simulink model "ModeSwitching"  (R2024a)
settings: Solver=FixedStepAuto  StartTime=0.0  StopTime=20  FixedStep=0.0005  RelTol=1e-3
values from neighbouring files (symbols this model uses):
  efficiency_map = efficiency_map / 100    [ModeSwitching_para.m]
  radius = 0.527    [ModeSwitching_para.m]
  s_thr = 0.2    [ModeSwitching_para.m]
  speed_rpm = [500,1000,1500,2000,2500,3000,3500,4000,4500,5000,5500,6000,6500,7000,7500,8000,8500,9000,9500,10000,10500,11000,11500,12000]    [ModeSwitching_para.m]
  torque_nm = [-600	-590	-580	-570	-560	-550	-540	-530	-520	-510	-500	-490	-480	-470	-460	-450	-440	-430	-420	-410	-400	-390	-380	-370	-360	-350	-340	-330	-320	-310	-300	-290	-280	-270	-260	-250	-240	-230	-220	-210	-200	-190	-180	-170	-160	-150	-140	-130	-120	-110	-100	-90	-80	-70	-60	-50	-40	-30	-20	-10	10	20	30	40	50	60	70	80	90	100	110	120	130	140	150	160	170	180	190	200	210	220	230	240	250	260	270	280	290	3 ...(+123 chars)    [ModeSwitching_para.m]
  v_min_s = 0.7    [ModeSwitching_para.m]
libraries: Solver_SF x1
(part 1 of 2)
settings Model: Creator=pan18  LastModifiedBy=pan18

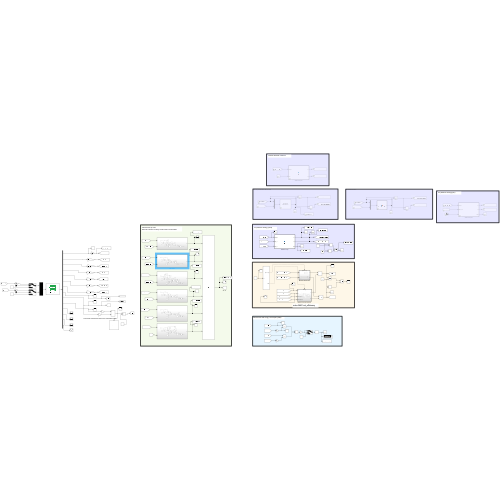
[thumbnail: Simulink's stored preview of the top-level diagram]
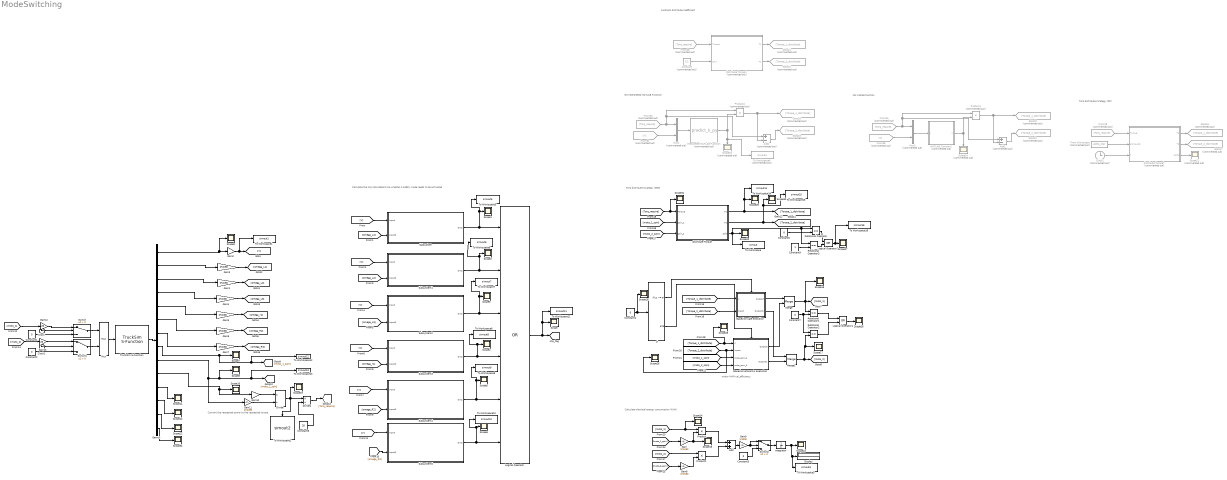
== system ModeSwitching ==
  note: NN matlab function
  note: NN Interpreted MATLAB Function
  note: Convert the requested power to the requested torque.
  note: Torq distribute strategy (GGS)
  note: Calculate the slip ratio
      | Determine whether a safety mode needs to be activated
  note: Calculate the total energy consumption (kWh)
  note: motor MAP-cal_efficiency
  note: constant distribute coefficient
  note: Torq distribute strategy (DP)
  Add : Sum
  Add1 : Sum  Commented=on  Inputs=+-
  Add2 : Sum  Commented=on  Inputs=+-
  Based on economic execution : Subsystem  TreatAsAtomicUnit=on
  Based on safe execution : Subsystem  TreatAsAtomicUnit=on
  Clock : Clock
  Clock1 : Clock
  Clock2 : Clock  Commented=on
  Constant : Constant  Commented=on  Value=0.2
  Constant{1..5,7} (6 alike) : Constant  Value=0
  Constant6 : Constant  Value=20
  Constant9 : Constant
  Demux : Demux  Outputs=14
  Display : Display
  Divide : Product  Inputs=*/
  Divide1 : Product  Inputs=*/
  From Workspace : FromWorkspace  Commented=on  VariableName=alpha_star
  From{28..30,34} (4 alike) : From  Commented=on  GotoTag=Torq_require
  From31 : From  Commented=on  GotoTag=V
  From35 : From  Commented=on  GotoTag=V
  Gain{,1,3..8,11} (9 alike) : Gain  Gain=2*pi/60
  Gain10 : Gain  Gain=1000
  Gain12 : Gain  Gain=20
  Gain13 : Gain  Gain=20
  Gain2 : Gain  Gain=1/3.6
  Gain9 : Gain  Gain=1/1000
  Goto{14,16,18,20} (4 alike) : Goto  Commented=on  GotoTag=Torque_1_distribute
  Goto{15,17,19,21} (4 alike) : Goto  Commented=on  GotoTag=Torque_2_distribute
  If : If  IfExpression=u1 ~= 0
  Integrator : Integrator
  Interpreted MATLAB Function : MATLABFcn  Commented=on  MATLABFcn=predict_k_py
  Logical Operator : Logic  Operator=OR  Inputs=6  AllPortsSameDT=off  OutDataTypeStr=boolean
  Logical Operator1 : Logic  Operator=OR  AllPortsSameDT=off  OutDataTypeStr=boolean
  Logical Operator2 : Logic  Operator=OR  AllPortsSameDT=off  OutDataTypeStr=boolean
  MATLAB Function1 : MATLAB Function  Commented=on  TreatAsAtomicUnit=on
  Merge : Merge
  Merge1 : Merge
  Mux : Mux  Inputs=2
  Mux1 : Mux  Commented=on  Inputs=2
  Mux3 : Mux  Commented=on  Inputs=2
  Product : Product
  Product1 : Product
  Product2 : Product  Commented=on
  Product4 : Product  Commented=on
  Relational Operator{,1..3} (4 alike) : RelationalOperator  Operator===  OutDataTypeStr=boolean  RndMeth=Simplest  InputSameDT=off
  Scope{,1..20,22,25..32} (30 alike) : Scope
  Scope21 : Scope  Commented=on
  Scope23 : Scope  Commented=on
  Scope24 : Scope  Commented=on
  Subsystem : Subsystem
  Subsystem1 : Subsystem
  Subsystem2 : Subsystem
  Subsystem3 : Subsystem
  Subsystem4 : Subsystem
  Subsystem6 : Subsystem
  Switch : Switch  Criteria=u2 > Threshold  SaturateOnIntegerOverflow=off  InputSameDT=off
  Switch1 : Switch  Criteria=u2 > Threshold  SaturateOnIntegerOverflow=off  InputSameDT=off
  Switch2 : Switch  Criteria=u2 > Threshold  SaturateOnIntegerOverflow=off  InputSameDT=off
  To Workspace : ToWorkspace  VariableName=simout  SaveFormat=Timeseries  SampleTime=-1
  To Workspace1 : ToWorkspace  VariableName=simout1  SaveFormat=Timeseries  SampleTime=-1
  To Workspace10 : ToWorkspace  VariableName=simout10  SaveFormat=Timeseries  SampleTime=-1
  To Workspace11 : ToWorkspace  VariableName=simout11  SaveFormat=Timeseries  SampleTime=-1
  To Workspace12 : ToWorkspace  VariableName=simout12  SaveFormat=Timeseries  SampleTime=-1
  To Workspace13 : ToWorkspace  VariableName=simout13  SaveFormat=Timeseries  SampleTime=-1
  To Workspace14 : ToWorkspace  VariableName=simout14  SaveFormat=Timeseries  SampleTime=-1
  To Workspace15 : ToWorkspace  VariableName=simout15  SaveFormat=Timeseries  SampleTime=-1
  To Workspace16 : ToWorkspace  VariableName=simout16  SaveFormat=Timeseries  SampleTime=-1
  To Workspace2 : ToWorkspace  VariableName=simout2  SaveFormat=Timeseries  SampleTime=-1
  To Workspace3 : ToWorkspace  VariableName=simout3  SaveFormat=Timeseries  SampleTime=-1
  To Workspace4 : ToWorkspace  Commented=on  VariableName=simout4  SaveFormat=Timeseries  SampleTime=-1
  To Workspace5 : ToWorkspace  VariableName=simout5  SaveFormat=Timeseries  SampleTime=-1
  To Workspace6 : ToWorkspace  VariableName=simout6  SaveFormat=Timeseries  SampleTime=-1
  To Workspace7 : ToWorkspace  VariableName=simout7  SaveFormat=Timeseries  SampleTime=-1
  To Workspace8 : ToWorkspace  VariableName=simout8  SaveFormat=Timeseries  SampleTime=-1
  To Workspace9 : ToWorkspace  VariableName=simout9  SaveFormat=Timeseries  SampleTime=-1
  TruckSim S-Function : Solver_SF/TruckSim S-Function  Priority=1  SIMFILE=simfile.sim  Run_RTs=off  vs_state_ind=Run  StopMode_ind=Vehicle Model
      settings: SourceProductName=TruckSim S-Function
  distribute Torque : MATLAB Function  TreatAsAtomicUnit=on
  distribute Torque1 : MATLAB Function  Commented=on  TreatAsAtomicUnit=on
  distribute Torque2 : MATLAB Function  Commented=on  TreatAsAtomicUnit=on
  wires:
  TruckSim S-Function/1 -> Demux/1
  Demux/1 -> Scope9/1, Gain2/1
  Demux/3 -> Gain1/1
  Gain2/1 -> To Workspace1/1, [V]
  Gain1/1 -> [omega_L2]
  Gain3/1 -> [omega_L1]
  Demux/2 -> Gain3/1
  Demux/4 -> Gain4/1
  Gain4/1 -> [omega_L3]
  Demux/5 -> Gain5/1
  Demux/6 -> Gain6/1
  Demux/7 -> Gain7/1
  Gain5/1 -> [omega_r1]
  Gain6/1 -> [omega_R2]
  Gain7/1 -> [omega_R3]
  [V] -> Subsystem/1(Inport)
  [omega_L1] -> Subsystem/2(Inport2)
  [omega_L2] -> Subsystem1/2(Inport2)
  [V] -> Subsystem1/1(Inport)
  [V] -> Subsystem2/1(Inport)
  [omega_L3] -> Subsystem2/2(Inport2)
  [V] -> Subsystem3/1(Inport)
  [V] -> Subsystem4/1(Inport)
  [omega_r1] -> Subsystem3/2(Inport2)
  [omega_R2] -> Subsystem4/2(Inport2)
  [V] -> Subsystem6/1(Inport)
  [omega_R3] -> Subsystem6/2(Inport2)
  Subsystem/1(Out1) -> To Workspace5/1, Scope1/1, Logical Operator/1
  Subsystem1/1(Out1) -> To Workspace6/1, Scope2/1, Logical Operator/2
  Subsystem3/1(Out1) -> To Workspace8/1, Scope4/1, Logical Operator/4
  Subsystem4/1(Out1) -> To Workspace9/1, Scope5/1, Logical Operator/5
  Logical Operator/1 -> To Workspace11/1, Scope/1, [Slip_tag]
  Subsystem2/1(Out1) -> To Workspace7/1, Scope3/1, Logical Operator/3
  Subsystem6/1(Out1) -> To Workspace10/1, Scope6/1, Logical Operator/6
  Constant1/1 -> Switch/3
  Constant2/1 -> Switch1/3
  Clock/1 -> Switch/2
  Clock1/1 -> Switch1/2
  [moto_1] -> Gain12/1
  [moto_2] -> Gain13/1
  If/1 -> Based on safe execution/Action
  If/2 -> Based on economic execution/Action
  Based on safe execution/1(Outport) -> Merge/1
  Based on economic execution/1(Outport) -> Merge/2
  Based on safe execution/2(Outport1) -> Merge1/1
  Based on economic execution/2(Outport1) -> Merge1/2
  Merge/1 -> Scope16/1, Relational Operator1/1, [moto_1]
  Merge1/1 -> Relational Operator2/2, Scope17/1, [moto_2]
  Demux/9 -> To Workspace13/1, [moto_2_spin], Scope8/1, Gain11/1
  [moto_1_spin] -> distribute Torque/2(spin_1)
  distribute Torque/1(T1) -> To Workspace14/1, Scope29/1, [Torque_1_distribute]
  distribute Torque/2(T2) -> Scope30/1, To Workspace15/1, [Torque_2_distribute]
  Demux/10 -> Gain10/1, Scope10/1
  Demux/11 -> Scope11/1
  Demux/12 -> Scope12/1
  [Torq_require] -> Scope31/1, distribute Torque/1(Torque)
  [Torque_1_distribute] -> Scope25/1, Based on economic execution/1(u)
  [Torque_2_distribute] -> Scope26/1, Based on economic execution/2(Inport)
  [moto_1_spin] -> Based on economic execution/3(moto_spin_1)
  [moto_2_spin] -> Based on economic execution/4(moto_spin_2)
  [Torque_2_distribute] -> Based on safe execution/2(Inport)
  [Torque_1_distribute] -> Based on safe execution/1(u)
  Switch1/1 -> Mux/2
  Switch/1 -> Mux/1
  [moto_1_spin] -> Gain/1
  [moto_2_spin] -> Gain8/1
  [moto_1] -> Scope14/1, Product/1
  Gain/1 -> Scope15/1, Product/2
  [moto_2] -> Product1/1
  Gain8/1 -> Product1/2
  Product/1 -> Add/1
  Product1/1 -> Add/2
  Add/1 -> Gain9/1
  Integrator/1 -> To Workspace3/1, Display/1, Scope13/1
  [moto_2_spin] -> distribute Torque/3(spin_2)
  Gain10/1 -> Divide/1
  Divide/1 -> Divide1/1, To Workspace2/1, Scope19/1
  Gain11/1 -> Divide/2
  Constant/1 -> distribute Torque1/2(split)
  distribute Torque1/1(T1) -> Goto14/1
  From28/1 -> distribute Torque1/1(Torque)
  distribute Torque1/2(T2) -> Goto15/1
  Constant4/1 -> Scope18/1, If/1
  distribute Torque/3(split) -> Relational Operator3/1, Relational Operator/1, Scope20/1, To Workspace/1
  Mux/1 -> TruckSim S-Function/1
  distribute Torque2/1(T1) -> Goto16/1
  From Workspace/1 -> distribute Torque2/2(alpha_star)
  From29/1 -> distribute Torque2/1(Torque)
  distribute Torque2/2(T2) -> Goto17/1
  Clock2/1 -> distribute Torque2/3(t)
  distribute Torque2/3(alpha) -> Scope21/1
  From30/1 -> Product2/1, Add1/1, Mux1/1
  Mux1/1 -> Interpreted MATLAB Function/1
  From31/1 -> Mux1/2
  Interpreted MATLAB Function/1 -> To Workspace4/1, Scope23/1, Product2/2
  Product2/1 -> Goto18/1, Add1/2
  Add1/1 -> Goto19/1
  Product4/1 -> Goto20/1, Add2/2
  MATLAB Function1/1(k) -> Scope24/1, Product4/2
  Add2/1 -> Goto21/1
  Mux3/1 -> MATLAB Function1/1(u)
  From34/1 -> Product4/1, Add2/1, Mux3/1
  From35/1 -> Mux3/2
  Demux/13 -> Scope22/1
  Gain9/1 -> Switch2/1, Switch2/2
  Switch2/1 -> Integrator/1
  Constant3/1 -> Switch2/3
  Constant5/1 -> Relational Operator/2
  Constant6/1 -> Divide1/2
  Divide1/1 -> [Torq_require]
  Gain12/1 -> Switch/1
  Gain13/1 -> Switch1/1
  Constant7/1 -> Relational Operator2/1, Relational Operator1/2
  Relational Operator1/1 -> Logical Operator1/1
  Logical Operator1/1 -> Scope28/1
  Constant9/1 -> Relational Operator3/2
  Relational Operator/1 -> Logical Operator2/1
  Relational Operator3/1 -> Logical Operator2/2
  Logical Operator2/1 -> To Workspace16/1, Scope27/1
  Relational Operator2/1 -> Logical Operator1/2
  Demux/8 -> [moto_1_spin], To Workspace12/1, Scope7/1
  Demux/14 -> Scope32/1

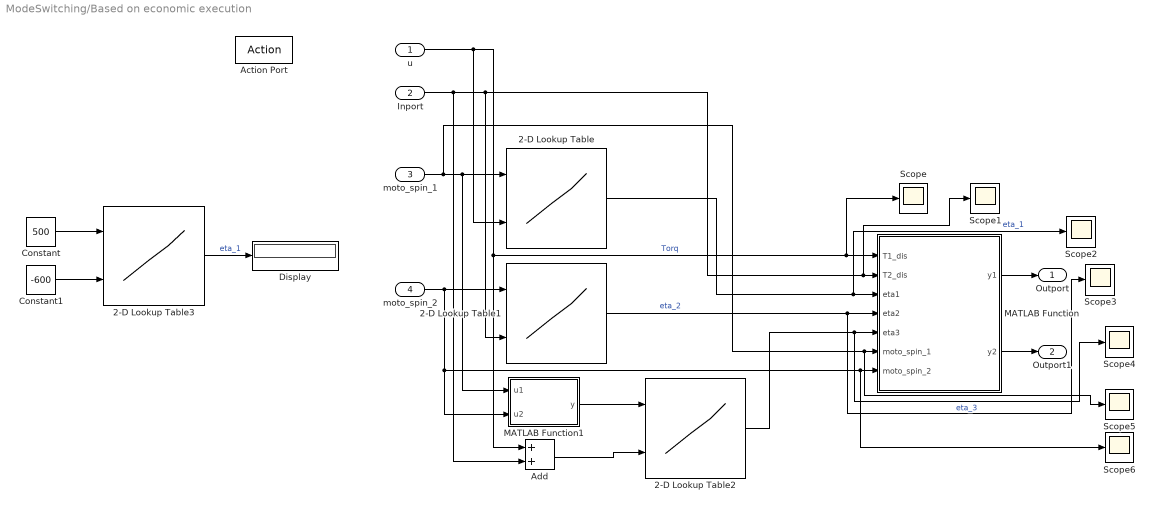
== system ModeSwitching/Based on economic execution ==
  u : Inport
  Inport : Inport  Port=2
  moto_spin_1 : Inport  Port=3
  moto_spin_2 : Inport  Port=4
  Action Port : ActionPort  ActionPortLabel=else
  2-D Lookup Table{,1..3} (4 alike) : Lookup_n-D  BreakpointsForDimension1=speed_rpm  BreakpointsForDimension2=torque_nm  Table=efficiency_map  InternalRulePriority=Speed  RndMeth=Simplest
      settings: InputPortMap=u0,u1
  Add : Sum
  Constant : Constant  Value=500
  Constant1 : Constant  Value=-600
  Display : Display
  MATLAB Function : MATLAB Function  TreatAsAtomicUnit=on
  MATLAB Function1 : MATLAB Function  TreatAsAtomicUnit=on
  Scope{,1..6} (7 alike) : Scope
  Outport : Outport
  Outport1 : Outport  Port=2
  wires:
  moto_spin_1/1 -> MATLAB Function1/1(u1), 2-D Lookup Table/1, Scope5/1, MATLAB Function/6(moto_spin_1)
  MATLAB Function/1(y1) -> Outport/1
  u/1 -> Scope/1, MATLAB Function/1(T1_dis), Add/1, 2-D Lookup Table/2  "Torq"
  Inport/1 -> Scope1/1, MATLAB Function/2(T2_dis), 2-D Lookup Table1/2, Add/2
  Add/1 -> 2-D Lookup Table2/2
  MATLAB Function1/1(y) -> 2-D Lookup Table2/1
  moto_spin_2/1 -> MATLAB Function1/2(u2), Scope6/1, MATLAB Function/7(moto_spin_2), 2-D Lookup Table1/1
  2-D Lookup Table/1 -> Scope2/1, MATLAB Function/3(eta1)  "eta_1"
  2-D Lookup Table1/1 -> Scope3/1, MATLAB Function/4(eta2)  "eta_2"
  2-D Lookup Table2/1 -> Scope4/1, MATLAB Function/5(eta3)  "eta_3"
  MATLAB Function/2(y2) -> Outport1/1
  Constant/1 -> 2-D Lookup Table3/1
  Constant1/1 -> 2-D Lookup Table3/2
  2-D Lookup Table3/1 -> Display/1  "eta_1"

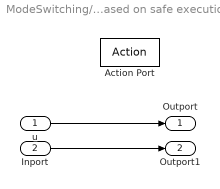
== system ModeSwitching/Based on safe execution ==
  u : Inport
  Inport : Inport  Port=2
  Action Port : ActionPort  ActionPortLabel=if(u1 ~= 0)
  Outport : Outport
  Outport1 : Outport  Port=2
  wires:
  Inport/1 -> Outport1/1
  u/1 -> Outport/1

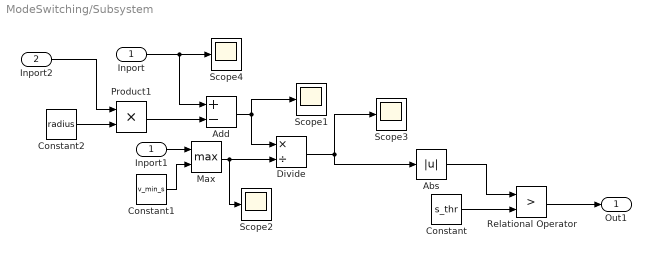
== system ModeSwitching/Subsystem ==
  Inport : Inport
  Inport2 : Inport  Port=2
  Abs : Abs  SaturateOnIntegerOverflow=off
  Add : Sum  Inputs=+-
  Constant : Constant  Value=s_thr
  Constant1 : Constant  Value=v_min_s
  Constant2 : Constant  Value=radius
  Divide : Product  Inputs=*/
  Inport1 : InportShadow
  Max : MinMax  Function=max  Inputs=2
  Product1 : Product
  Relational Operator : RelationalOperator  Operator=>  OutDataTypeStr=boolean  InputSameDT=off
  Scope{1..4} (4 alike) : Scope
  Out1 : Outport
  wires:
  Constant/1 -> Relational Operator/2
  Constant2/1 -> Product1/2
  Inport/1 -> Scope4/1, Add/1
  Inport2/1 -> Product1/1
  Add/1 -> Divide/1, Scope1/1
  Divide/1 -> Abs/1, Scope3/1
  Product1/1 -> Add/2
  Relational Operator/1 -> Out1/1
  Max/1 -> Scope2/1, Divide/2
  Inport1/1 -> Max/1
  Constant1/1 -> Max/2
  Abs/1 -> Relational Operator/1

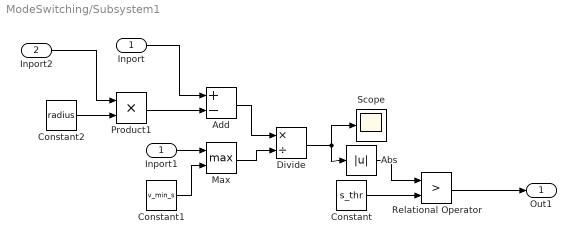
== system ModeSwitching/Subsystem1 ==
  Inport : Inport
  Inport2 : Inport  Port=2
  Abs : Abs  SaturateOnIntegerOverflow=off
  Add : Sum  Inputs=+-
  Constant : Constant  Value=s_thr
  Constant1 : Constant  Value=v_min_s
  Constant2 : Constant  Value=radius
  Divide : Product  Inputs=*/
  Inport1 : InportShadow
  Max : MinMax  Function=max  Inputs=2
  Product1 : Product
  Relational Operator : RelationalOperator  Operator=>  OutDataTypeStr=boolean  InputSameDT=off
  Scope : Scope
  Out1 : Outport
  wires:
  Constant/1 -> Relational Operator/2
  Constant2/1 -> Product1/2
  Inport/1 -> Add/1
  Inport2/1 -> Product1/1
  Add/1 -> Divide/1
  Divide/1 -> Scope/1, Abs/1
  Product1/1 -> Add/2
  Relational Operator/1 -> Out1/1
  Inport1/1 -> Max/1
  Max/1 -> Divide/2
  Constant1/1 -> Max/2
  Abs/1 -> Relational Operator/1

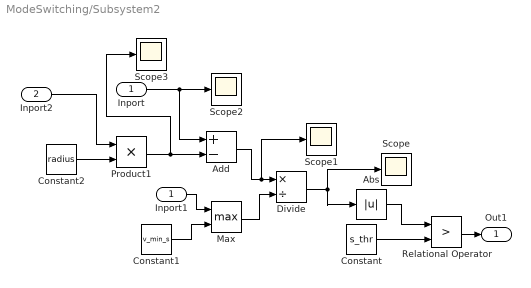
== system ModeSwitching/Subsystem2 ==
  Inport : Inport
  Inport2 : Inport  Port=2
  Abs : Abs  SaturateOnIntegerOverflow=off
  Add : Sum  Inputs=+-
  Constant : Constant  Value=s_thr
  Constant1 : Constant  Value=v_min_s
  Constant2 : Constant  Value=radius
  Divide : Product  Inputs=*/
  Inport1 : InportShadow
  Max : MinMax  Function=max  Inputs=2
  Product1 : Product
  Relational Operator : RelationalOperator  Operator=>  OutDataTypeStr=boolean  InputSameDT=off
  Scope{,1..3} (4 alike) : Scope
  Out1 : Outport
  wires:
  Relational Operator/1 -> Out1/1
  Product1/1 -> Scope3/1, Add/2
  Divide/1 -> Scope/1, Abs/1
  Add/1 -> Scope1/1, Divide/1
  Inport2/1 -> Product1/1
  Inport/1 -> Add/1, Scope2/1
  Constant2/1 -> Product1/2
  Constant/1 -> Relational Operator/2
  Constant1/1 -> Max/2
  Inport1/1 -> Max/1
  Max/1 -> Divide/2
  Abs/1 -> Relational Operator/1

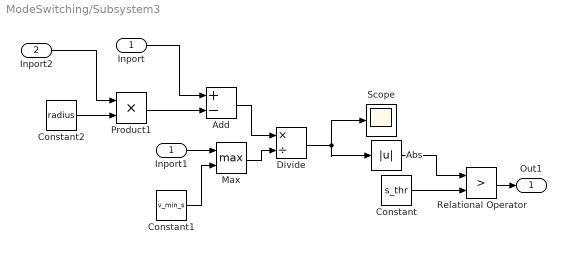
== system ModeSwitching/Subsystem3 ==
  Inport : Inport
  Inport2 : Inport  Port=2
  Abs : Abs  SaturateOnIntegerOverflow=off
  Add : Sum  Inputs=+-
  Constant : Constant  Value=s_thr
  Constant1 : Constant  Value=v_min_s
  Constant2 : Constant  Value=radius
  Divide : Product  Inputs=*/
  Inport1 : InportShadow
  Max : MinMax  Function=max  Inputs=2
  Product1 : Product
  Relational Operator : RelationalOperator  Operator=>  OutDataTypeStr=boolean  InputSameDT=off
  Scope : Scope
  Out1 : Outport
  wires:
  Constant/1 -> Relational Operator/2
  Constant2/1 -> Product1/2
  Inport/1 -> Add/1
  Inport2/1 -> Product1/1
  Add/1 -> Divide/1
  Divide/1 -> Abs/1, Scope/1
  Product1/1 -> Add/2
  Relational Operator/1 -> Out1/1
  Inport1/1 -> Max/1
  Max/1 -> Divide/2
  Constant1/1 -> Max/2
  Abs/1 -> Relational Operator/1

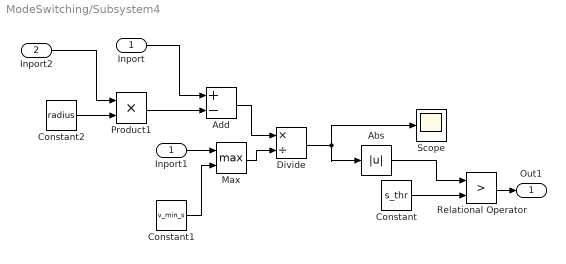
== system ModeSwitching/Subsystem4 ==
  Inport : Inport
  Inport2 : Inport  Port=2
  Abs : Abs  SaturateOnIntegerOverflow=off
  Add : Sum  Inputs=+-
  Constant : Constant  Value=s_thr
  Constant1 : Constant  Value=v_min_s
  Constant2 : Constant  Value=radius
  Divide : Product  Inputs=*/
  Inport1 : InportShadow
  Max : MinMax  Function=max  Inputs=2
  Product1 : Product
  Relational Operator : RelationalOperator  Operator=>  OutDataTypeStr=boolean  InputSameDT=off
  Scope : Scope
  Out1 : Outport
  wires:
  Relational Operator/1 -> Out1/1
  Product1/1 -> Add/2
  Divide/1 -> Abs/1, Scope/1
  Add/1 -> Divide/1
  Inport2/1 -> Product1/1
  Inport/1 -> Add/1
  Constant2/1 -> Product1/2
  Constant/1 -> Relational Operator/2
  Constant1/1 -> Max/2
  Max/1 -> Divide/2
  Inport1/1 -> Max/1
  Abs/1 -> Relational Operator/1

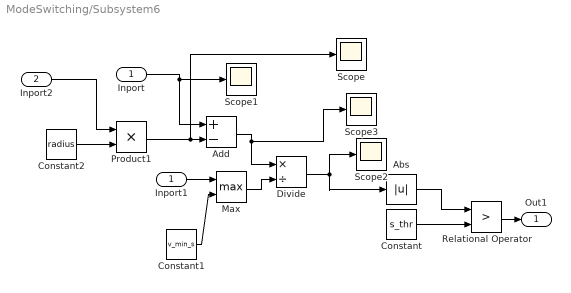
== system ModeSwitching/Subsystem6 ==
  Inport : Inport
  Inport2 : Inport  Port=2
  Abs : Abs  SaturateOnIntegerOverflow=off
  Add : Sum  Inputs=+-
  Constant : Constant  Value=s_thr
  Constant1 : Constant  Value=v_min_s
  Constant2 : Constant  Value=radius
  Divide : Product  Inputs=*/
  Inport1 : InportShadow
  Max : MinMax  Function=max  Inputs=2
  Product1 : Product
  Relational Operator : RelationalOperator  Operator=>  OutDataTypeStr=boolean  InputSameDT=off
  Scope{,1..3} (4 alike) : Scope
  Out1 : Outport
  wires:
  Relational Operator/1 -> Out1/1
  Product1/1 -> Scope/1, Add/2
  Divide/1 -> Scope2/1, Abs/1
  Add/1 -> Divide/1, Scope3/1
  Inport2/1 -> Product1/1
  Inport/1 -> Add/1, Scope1/1
  Constant2/1 -> Product1/2
  Constant/1 -> Relational Operator/2
  Constant1/1 -> Max/2
  Inport1/1 -> Max/1
  Max/1 -> Divide/2
  Abs/1 -> Relational Operator/1

== matlab function ModeSwitching/distribute Torque ==
  data: Torque input; T1 output; spin_1 input; T2 output; spin_2 input; split output
function [T1, T2, split] = fcn(Torque, spin_1, spin_2)

    % speed_rpm = [0,1000,2000,3000,4000,5000,6000,7000,8000];
    % torque_nm = [0,50,100,150,200,250,300];
    % 
    % efficiency_map = [
    %     0.00,0.00,0.00,0.00,0.00,0.00,0.00;
    %     0.70,0.85,0.88,0.90,0.89,0.87,0.85;
    %     0.75,0.88,0.91,0.92,0.91,0.90,0.88;
    %     0.80,0.90,0.92,0.93,0.92,0.91,0.89;
    %     0.82,0.91,0.93,0.94,0.93,0.92,0.90;
    %     0.83,0.92,0.94,0.94,0.93,0.92,0.90;
    %     0.82,0.91,0.93,0.93,0.92,0.91,0.89;
    %     0.80,0.89,0.91,0.91,0.90,0.88,0.86;
    %     0.75,0.85,0.87,0.87,0.86,0.84,0.82
    % ];
    
        speed_rpm = [500,1000,1500,2000,2500,3000,3500,4000,4500,5000,5500,6000,6500,7000,7500,8000,8500,9000,9500,10000,10500,11000,11500,12000];
        torque_nm = [-600	-590	-580	-570	-560	-550	-540	-530	-520	-510	-500	-490	-480	-470	-460	-450	-440	-430	-420	-410	-400	-390	-380	-370	-360	-350	-340	-330	-320	-310	-300	-290	-280	-270	-260	-250	-240	-230	-220	-210	-200	-190	-180	-170	-160	-150	-140	-130	-120	-110	-100	-90	-80	-70	-60	-50	-40	-30	-20	-10	10	20	30	40	50	60	70	80	90	100	110	120	130	140	150	160	170	180	190	200	210	220	230	240	250	260	270	280	290	300	310	320	330	340	350	360	370	380	390	400	410	420	430	440	450	460	470	480	490	500	510	520	530	540	550	560	570	580	590	600];
    
        efficiency_map = [
    43.53935193	44.38180165	45.2135057	46.03470163	46.84559756	47.64646587	48.43810692	49.21992322	49.99284637	50.75734642	51.51392029	52.26311414	53.00550814	53.74170179	54.47231871	55.19800339	55.91949984	56.63730548	57.3522004	58.06532088	58.77483708	59.48160724	60.18442643	60.87971856	61.56903426	62.25151104	62.92502023	63.59027539	64.24625445	64.89434608	65.53331607	66.16350166	66.78543615	67.39981079	68.00759963	68.61011156	69.20855047	69.80395362	70.39719416	70.98897735	71.57983657	72.17006769	72.7599515	73.34946925	73.93848871	74.52673858	75.11378469	75.69939688	76.28099795	76.85831842	77.42861376	77.98804952	78.52982996	79.04314263	79.50806881	79.88619503	80.09632293	79.94102844	78.8154095	73.64688876	84.13036773	88.51802035	89.52055938	89.61050076	89.35428458	88.94106936	88.45132806	87.92399376	87.37985563	86.82985899	86.28065493	85.73587588	85.1976707	84.66864939	84.14738875	83.63485228	83.13105256	82.6358164	82.14880915	81.669502	81.1975077	80.7320996	80.27257068	79.81815419	79.36803012	78.9213298	78.47714387	78.03466606	77.59448788	77.15425574	76.7146919	76.27569495	75.83642928	75.39924707	74.96151364	74.52543029	74.09161393	73.65883365	73.22823979	72.80032504	72.37569731	71.95466022	71.53719287	71.122699	70.71090606	70.30148986	69.89416001	69.48863633	69.08466116	68.68200048	68.2804546	67.87983957	67.48045839	67.08130422	66.68268353	66.28452163	65.886774	65.48942603	65.09249369	64.69603571;
    70.70395181	71.12828879	71.54733523	71.9611718	72.36988248	72.77358326	73.17240133	73.56655489	73.95620165	74.34155549	74.72284785	75.10032688	75.47425589	75.84491076	76.21257855	76.57755237	76.94017583	77.30067773	77.65950426	78.01673289	78.37231074	78.72579431	79.07654248	79.423738	79.76721116	80.1065528	80.4412103	80.7711058	81.09594765	81.41586288	81.73065047	82.04041286	82.34534066	82.64571008	82.94194286	83.23461642	83.52424276	83.81123521	84.09590363	84.37844636	84.65893999	84.93732131	85.21338655	85.48676548	85.75690324	86.0230374	86.28413635	86.53883643	86.78506829	87.02026315	87.24051131	87.44003071	87.60991481	87.73581405	87.79317836	87.73671599	87.47393302	86.78504814	85.00845411	78.78732879	84.91416855	90.04430098	91.61374219	92.19689619	92.38577547	92.38126794	92.27077162	92.09799257	91.88724444	91.65230749	91.40205468	91.14197521	90.87576443	90.60703701	90.33584358	90.0639528	89.79218771	89.52109177	89.25097731	88.98193629	88.71410007	88.44729274	88.18131601	87.91589438	87.65068534	87.38528683	87.11924694	86.85215485	86.58475541	86.31506616	86.04384987	85.77108278	85.49604187	85.22038368	84.9430733	84.66478162	84.38640844	84.10669616	83.82669379	83.54671874	83.26653554	82.98837228	82.71041808	82.43278583	82.15539627	81.87807555	81.60066126	81.32299117	81.04491368	80.76628927	80.48700271	80.20694134	79.92651512	79.64468378	79.36183276	79.07791741	78.79291329	78.50683072	78.21965973	77.93146208;
    80.22627696	80.50883269	80.78786957	81.06341978	81.33552942	81.6042654	81.86954661	82.13183835	82.39105571	82.64732884	82.90080188	83.15162422	83.39995463	83.64596137	83.88981913	84.13171289	84.37182385	84.61031796	84.84724804	85.08318746	85.31776953	85.55046929	85.78091192	86.00907359	86.23426749	86.4562974	86.67512667	86.89040471	87.10205842	87.3098971	87.51399975	87.71439465	87.91116378	88.10444735	88.29447939	88.48158216	88.66602468	88.84799997	89.02761795	89.20489608	89.37974718	89.55197515	89.72120808	89.88694688	90.04848594	90.20488859	90.35491143	90.49680543	90.62863033	90.74703202	90.84767549	90.92406743	90.96650336	90.95931433	90.87617393	90.66909736	90.24107127	89.3632189	87.3507406	80.7275059	85.39254798	90.82266341	92.60967061	93.37828756	93.7340679	93.88330784	93.91634811	93.87878436	93.796258	93.68356026	93.5503434	93.40273056	93.24494786	93.08091518	92.91119795	92.7378223	92.56187709	92.38414184	92.20514435	92.02519047	91.84458742	91.66335847	91.48149283	91.29890159	91.11542926	90.93086233	90.74493951	90.55741674	90.36907895	90.1781335	89.98533746	89.79069173	89.59354578	89.3953666	89.19525132	88.99381329	88.79177561	88.58791276	88.38320931	88.17785015	87.97216205	87.76627922	87.56058015	87.35442007	87.1478384	86.94073044	86.73298953	86.524507	86.3151802	86.10491379	85.89363247	85.68125713	85.46823767	85.2535398	85.03757642	84.82031677	84.60174474	84.38188078	84.1606988	83.93825732;
    84.97238119	85.18393077	85.39283915	85.59911379	85.80278142	86.00388397	86.20223544	86.39842498	86.59224524	86.78378391	86.9731411	87.16041575	87.34571388	87.52914921	87.71083948	87.89091409	88.069474	88.24665132	88.42231313	88.59726502	88.77097105	88.94287884	89.11277246	89.28099637	89.44658484	89.60947796	89.76992262	89.92738612	90.0819002	90.233142	90.3813119	90.52639649	90.66841936	90.80744757	90.94361454	91.07710692	91.20806309	91.33655519	91.46258072	91.58605219	91.70678347	91.82449207	91.93869748	92.04880721	92.15400445	92.25322082	92.34505021	92.4274751	92.49853971	92.55435112	92.59018951	92.59894852	92.57014742	92.48686336	92.32090152	92.02117671	91.48492226	90.45622556	88.25772722	81.18712431	85.2526146	90.99274049	92.95615894	93.85564677	94.32036656	94.5653294	94.68507675	94.72756768	94.71992436	94.6779322	94.61195837	94.52865914	94.43268667	94.3282183	94.21615721	94.09872384	93.97718886	93.85248874	93.72529069	93.59603564	93.46514082	93.33275102	93.19896897	93.06381788	92.92725411	92.78917669	92.64943814	92.50789478	92.36535947	92.22015281	92.07303327	91.92401901	91.77251688	91.61984996	91.46523204	91.30925002	91.1524772	90.99378143	90.83398923	90.6733338	90.51199856	90.35008149	90.18812776	90.02535333	89.86189934	89.69770435	89.5326944	89.36679355	89.19992946	89.03203453	88.86305913	88.69294566	88.52217015	88.34970354	88.17597757	88.00097185	87.82467732	87.64712261	87.46827318	87.28818722;
    87.14124322	87.31244865	87.48152962	87.64847576	87.8132996	87.97602606	88.13640191	88.29509536	88.45182161	88.60664261	88.75963236	88.9108597	89.06040001	89.20833556	89.35475162	89.49974581	89.64337449	89.78575118	89.92664017	90.06699488	90.20613003	90.34350526	90.47898223	90.61309722	90.74468944	90.87378269	91.00080513	91.1250595	91.24662741	91.36511059	91.48076037	91.59352438	91.70337827	91.81033256	91.91444994	92.01582918	92.11452083	92.21051069	92.30370979	92.39394247	92.48093069	92.56429906	92.64344866	92.71766513	92.78598177	92.84714656	92.89952207	92.94075382	92.96866701	92.97872347	92.96555463	92.92108002	92.83345509	92.68359209	92.43982761	92.04498178	91.38432618	90.17318154	87.65637092	79.71439976	83.79564003	90.0795463	92.29789866	93.35785685	93.9403674	94.27955896	94.47881799	94.59081338	94.64544431	94.66025008	94.64678568	94.61255779	94.56280118	94.50214927	94.43190054	94.35454462	94.27158095	94.18413505	94.09303379	93.9988615	93.90214942	93.80315659	93.70208707	93.59905868	93.4941175	93.38724888	93.2783894	93.16747084	93.05533248	92.94039291	92.82342093	92.7035714	92.58298138	92.46019131	92.33543015	92.20928363	92.08219396	91.9531385	91.82288568	91.6916425	91.55985702	91.42665492	91.29369011	91.15970054	91.0249179	90.88931006	90.75282348	90.6154039	90.47699949	90.33756195	90.19705999	90.05545158	89.91322931	89.76937533	89.62433398	89.47809464	89.33065603	89.18205538	89.0322565	88.88132081;
    89.12519451	89.26759127	89.40821141	89.54703388	89.68406297	89.81893515	89.95248379	90.08430126	90.21442574	90.34290114	90.46978298	90.59511808	90.7189595	90.84136615	90.9623989	91.08213074	91.20058552	91.31786042	91.43365213	91.54900756	91.66311825	91.7755053	91.88608232	91.99507281	92.10252219	92.20756668	92.31015286	92.41052473	92.50845165	92.60350804	92.69598003	92.78579442	92.87289935	92.95727064	93.03892329	93.11789249	93.19416626	93.26767055	93.33825848	93.40569774	93.46965392	93.52969837	93.5851644	93.63527347	93.67898064	93.71493936	93.74139346	93.75580728	93.75593614	93.73687945	93.69295546	93.6155985	93.49230403	93.30293085	93.01416317	92.56596847	91.83811873	90.5332346	87.86080912	79.51470957	83.47516072	90.0191001	92.36717526	93.51233465	94.15978393	94.55248036	94.79796346	94.95115152	95.04329918	95.09279672	95.11179399	95.10782148	95.0880616	95.05485127	95.01140745	94.95992333	94.90201788	94.83891649	94.77153146	94.70052686	94.62649888	94.54977387	94.47061807	94.38920941	94.30565293	94.21999246	94.13222304	94.04232822	93.95117355	93.85721792	93.76124178	93.66242996	93.56289746	93.46114279	93.35747289	93.25247523	93.14645388	93.03847842	92.92925722	92.8189722	92.70802739	92.59552326	92.48322153	92.36975903	92.25542759	92.1402198	92.02409771	91.90702393	91.78896251	91.6698799	91.54975904	91.4285693	91.30682378	91.18349708	91.05904991	90.93347834	90.80678615	90.67901669	90.55013029	90.42019012;
    90.52961537	90.65143374	90.77172244	90.89045221	91.00762094	91.12282686	91.23695764	91.3495608	91.46066227	91.57029254	91.67849357	91.78529563	91.8907353	91.99485423	92.09769526	92.19931283	92.29970757	92.39896396	92.49673425	92.59412801	92.69003964	92.78463916	92.87729176	92.9684855	93.05820445	93.14567818	93.23083938	93.31394856	93.39476283	93.47284807	93.54850786	93.62165136	93.69220425	93.76011421	93.82535813	93.88792134	93.94774211	94.00469772	94.05859305	94.10914725	94.15597607	94.19860194	94.23629537	94.26821573	94.29324167	94.30993351	94.31641743	94.3099838	94.28829644	94.24610803	94.17741498	94.07315805	93.9201461	93.69714648	93.36910506	92.87295389	92.08254976	90.68684464	87.85638711	79.08140005	83.04076584	89.8507913	92.32659264	93.55205225	94.25842845	94.69817449	94.98327619	95.17104017	95.29414645	95.37186736	95.41696372	95.43739127	95.4406528	95.42929703	95.4067338	95.37529683	95.33671941	95.29232107	95.24309347	95.18977308	95.13301495	95.07320425	95.01066088	94.94561384	94.8782174	94.80856356	94.73669497	94.66263736	94.58728313	94.5091166	94.4289329	94.3459406	94.26224613	94.17629694	94.0884833	93.9994021	93.90921673	93.81709983	93.72370217	93.62918937	93.53391469	93.43700031	93.34027473	93.24227903	93.14336218	93.04353752	92.94277886	92.84106212	92.73836397	92.63466264	92.52995266	92.42421241	92.3179745	92.21020239	92.10137277	91.99148745	91.88055478	91.76862363	91.65565188	91.54170492;
    91.57169516	91.67808126	91.78312167	91.88678041	91.98905021	92.08949768	92.18905614	92.28723614	92.38405398	92.47952962	92.57369456	92.66656583	92.75816728	92.84852708	92.93767399	93.02564766	93.11243143	93.19809924	93.28227415	93.36610409	93.44840138	93.52940385	93.60849561	93.68621683	93.76247191	93.83661402	93.90855034	93.97853712	94.04632182	94.11147375	94.1743028	94.23470251	94.29257925	94.34785666	94.40047951	94.45039181	94.49749011	94.54161004	94.58251425	94.61987841	94.6532726	94.682173	94.70579044	94.72322352	94.73327562	94.73441484	94.72465034	94.70110314	94.66133225	94.59975315	94.51003523	94.38262065	94.20361523	93.95067164	93.58694448	93.04621762	92.19617569	90.71152014	87.72157491	78.50238074	82.53884867	89.61591117	92.21745546	93.5198048	94.28112941	94.76371997	95.08416458	95.30223329	95.45206968	95.55384429	95.62093742	95.6617304	95.68405339	95.69065769	95.6851445	95.66998516	95.64702381	95.61767052	95.58294599	95.54379339	95.50078376	95.4544019	95.40501592	95.35289996	95.29825122	95.24120315	95.1818389	95.12022004	95.05726639	94.99147751	94.92366524	94.85305793	94.78176224	94.7081673	94.63275198	94.55614925	94.47761828	94.39859271	94.31756124	94.23537367	94.1523257	94.06759906	93.98305582	93.8971463	93.81027482	93.72247299	93.63372371	93.54401386	93.45333049	93.3616616	93.26901153	93.175366	93.08127658	92.98569274	92.88910702	92.79152628	92.69296295	92.59347103	92.49300654	92.39163736;
    92.37215385	92.46653946	92.55972141	92.65165802	92.74233763	92.83129967	92.91951735	93.0064695	93.09216453	93.17661377	93.25984032	93.34185026	93.42265711	93.50227811	93.58073059	93.6580419	93.73418205	93.80921589	93.88274818	93.9559433	94.02707406	94.09788819	94.16633042	94.23346125	94.29909784	94.36273686	94.42425095	94.48387696	94.54135549	94.59626755	94.64892164	94.69919707	94.74698298	94.79218168	94.83470982	94.87447582	94.91133986	94.94510056	94.97548239	95.00212092	95.02454334	95.04218139	95.05418826	95.0596027	95.05715358	95.04521737	95.02168665	94.98351626	94.92815172	94.84967739	94.7414324	94.59335725	94.39084384	94.1104152	93.71340012	93.13036037	92.22263969	90.65032187	87.49996725	77.82649098	81.99540848	89.33763394	92.06296435	93.43964304	94.2530958	94.77560869	95.12845053	95.37389376	95.54756557	95.67054237	95.75682797	95.81522856	95.85390559	95.87580633	95.88472209	95.88325967	95.8733716	95.85655593	95.83390674	95.80642943	95.77474956	95.73940077	95.70079556	95.65924916	95.61499736	95.56821043	95.51900706	95.46748031	95.41457785	95.35880722	95.3009984	95.24039695	95.17911558	95.1154792	95.05006051	94.98355638	94.91496655	94.84551959	94.77482247	94.70255493	94.62932549	94.5544112	94.47967576	94.40348463	94.32629648	94.24815945	94.1690637	94.08900537	94.00798032	93.92598488	93.84303193	93.75911333	93.67479925	93.58902302	93.5022929	93.4146203	93.32602139	93.23655492	93.14617544	93.05495343;
    93.00345013	93.08826115	93.17193398	93.25449325	93.33589936	93.41566771	93.49480728	93.57276889	93.64955425	93.72516747	93.79962466	93.87292248	93.94506589	94.01606295	94.08592141	94.15465804	94.22223238	94.28870113	94.35365912	94.41819637	94.48085513	94.54296071	94.60279289	94.66134928	94.71835995	94.7734851	94.82653776	94.87773208	94.92681149	94.97337001	95.01770903	95.05969463	95.09920018	95.13610858	95.17031113	95.2016847	95.2300568	95.25519236	95.27678047	95.29441901	95.30759415	95.31569454	95.31781712	95.31294143	95.29972243	95.27644533	95.24088639	95.18983672	95.12062229	95.02700042	94.90197801	94.73499184	94.5107125	94.20452335	93.77590381	93.15214309	92.18812808	90.52908656	87.21772111	77.08303492	81.4260925	89.02996342	91.87715158	93.3261214	94.18959089	94.74988909	95.1329971	95.4037068	95.599138	95.74127538	95.84474756	95.91878419	95.97187998	96.00717311	96.02864393	96.03903292	96.04039914	96.0343267	96.02198086	96.00442748	95.98234413	95.95631072	95.92678145	95.89410972	95.85856677	95.82035633	95.77962909	95.73650644	95.69196424	95.64451261	95.59500078	95.54268982	95.48970239	95.43429414	95.37713693	95.31898919	95.25858699	95.19723168	95.13487583	95.07078429	95.00562333	94.93879897	94.87214597	94.80395145	94.7347277	94.66453828	94.59337918	94.52125459	94.44816804	94.37412313	94.29946322	94.22363449	94.14680304	94.06925842	93.99063585	93.91111622	93.83071691	93.74946689	93.66738846	93.5845245;
    93.51167496	93.5886281	93.66455333	93.73942682	93.81322997	93.8859487	93.95757333	94.02809747	94.09751952	94.16584295	94.23307371	94.29916631	94.36424543	94.4281917	94.49087233	94.55251901	94.61304682	94.67191757	94.73072127	94.78783857	94.8437343	94.89827236	94.95097893	95.00242512	95.05225989	95.10032521	95.14633462	95.19050365	95.23257126	95.27214869	95.3095258	95.34455619	95.37709854	95.40701771	95.43418169	95.45843872	95.47958637	95.49735824	95.51141014	95.52130393	95.52648622	95.52630349	95.51979751	95.50588904	95.48315951	95.44980325	95.40348035	95.34082005	95.25902447	95.15152675	95.01100025	94.82637678	94.58160033	94.25090774	93.79191257	93.12859578	92.10930522	90.36425594	86.89148198	76.29066111	80.84083839	88.70186601	91.66899977	93.18856243	94.10039594	94.69685015	95.10862023	95.40302049	95.61866537	95.77844678	95.8976177	95.98582938	96.05191045	96.09918603	96.13182441	96.15269831	96.16397181	96.16731353	96.16395827	96.15503095	96.14125925	96.12326748	96.10154949	96.07649465	96.04840734	96.01752222	95.98401933	95.94804604	95.91060665	95.87020982	95.82772473	95.78242701	95.73645179	95.68771216	95.63831146	95.58660778	95.53341552	95.47897515	95.42329907	95.36536832	95.30711307	95.24828174	95.18784953	95.12628242	95.06376694	95.0002763	94.93582623	94.87041954	94.80406272	94.73676439	94.66853423	94.59935637	94.52930729	94.45835859	94.38652642	94.31383105	94.24029749	94.16986762	94.09800214	94.02223441;
    0	0	0	0	0	94.27068858	94.34130398	94.40871857	94.47298839	94.53415761	94.59438378	94.64740927	94.70354486	94.76373925	94.82057671	94.87630334	94.93090825	94.98437832	95.0366975	95.08784254	95.13768775	95.18619499	95.23322669	95.2785955	95.32237818	95.36434943	95.40439865	95.44253523	95.47854281	95.51225358	95.54394156	95.57299724	95.59920084	95.62307942	95.64425393	95.66235351	95.6772275	95.68858195	95.69604089	95.6991315	95.69726189	95.68973707	95.6755444	95.65354624	95.62225083	95.5797618	95.52362322	95.45030404	95.35687929	95.23645995	95.08138506	94.8800807	94.61576039	94.26150974	93.77306463	93.07107199	91.99728087	90.16679126	86.53234693	75.46180232	80.24622584	88.38162382	91.44452346	93.03321268	93.99206794	94.62339198	95.06257607	95.37945073	95.61412219	95.79038643	95.92411906	96.02539077	96.10336388	96.16154719	96.20429592	96.23461365	96.25476825	96.26651162	96.27114674	96.2698565	96.2634172	96.25249609	96.23762509	96.21923227	96.19773124	96.17347655	96.14642176	96.11671644	96.08464946	96.05028812	96.01384822	95.97536397	95.93498504	95.89279779	95.84886714	95.80327235	95.75613524	95.7074695	95.65741408	95.59933699	95.55538935	95.50594855	95.4564259	95.4036197	95.34741591	95.28771355	95.22443534	95.15751072	95.08683711	95.0122457	94.93352792	94.85043175	94.76265262	94.66982058	94.57148231	0	0	0	0	0;
    0	0	0	0	0	0	0	0	0	94.65991647	94.74349437	94.82300555	94.89871374	94.97083386	95.03954274	95.1049836	95.16726978	95.22648728	95.28269857	95.33596058	95.3863236	95.43380582	95.47839873	95.5200674	95.55874871	95.59434896	95.62674123	95.65576029	95.68303085	95.7048388	95.73364029	95.75752849	95.77884312	95.79743225	95.81313869	95.82567261	95.83493325	95.84061193	95.84215776	95.83926876	95.83103504	95.81687163	95.79573043	95.76636808	95.72723345	95.67633971	95.61111492	95.52786913	95.42354781	95.29094125	95.12205375	94.90480516	94.62167577	94.24459662	93.72741737	92.98743205	91.85974665	89.94428117	86.13770737	74.60506618	79.64675573	88.03016853	91.20789937	92.8644137	93.86916645	94.5343145	94.99991393	95.33829877	95.591061	95.78289591	95.93029924	96.04375873	96.1327695	96.2010213	96.25305522	96.29200454	96.32023979	96.33957061	96.35133074	96.35687382	96.35708964	96.35255499	96.34385431	96.33149	96.3157469	96.29696884	96.27851129	96.2621312	96.242668	96.21844473	96.18982007	96.15706851	96.12039892	96.07996314	96.03586375	95.9881604	95.93687495	95.88199555	95.82348349	95.76128288	95.69530219	95.62543757	95.55155903	95.47349638	95.39103295	95.30389576	95.21174223	95.11414256	95.01055465	94.90029147	94.78248404	0	0	0	0	0	0	0	0	0;
    0	0	0	0	0	0	0	0	0	0	0	0	0	94.87713767	94.96774821	95.05341171	95.13450888	95.21134085	95.28414338	95.35309648	95.41833288	95.47995314	95.53807859	95.59281486	95.64422988	95.69235386	95.73717907	95.77868303	95.81683936	95.85159382	95.8828566	95.9104941	95.93431877	95.95407716	95.96943039	95.97992261	95.98499202	95.9839882	95.97614595	95.96053818	95.93677379	95.91545724	95.88790257	95.85172501	95.8053298	95.74667175	95.67311163	95.58035874	95.46571675	95.32150031	95.13937882	94.90676572	94.60540591	94.20607369	93.66072621	92.88329062	91.7021967	89.70214619	85.73213661	73.72660131	79.04558711	87.6714238	90.96211683	92.68527594	93.73495988	94.43305975	94.92425574	95.28336831	95.55346685	95.76014006	95.92050071	96.04545108	96.14462486	96.22247707	96.28305265	96.32997666	96.35654973	96.40198328	96.43489459	96.45629662	96.46783278	96.47080058	96.4662601	96.45511799	96.43813518	96.41592178	96.38895378	96.35755185	96.32193042	96.28222822	96.23852675	96.1908987	96.13938818	96.08398263	96.02461738	95.96117846	95.89350318	95.82137937	95.74455915	95.66283001	95.57593783	95.48353777	95.38517841	95.28032599	95.16830218	95.04819582	94.91877917	0	0	0	0	0	0	0	0	0	0	0	0	0;
    0	0	0	0	0	0	0	0	0	0	0	0	0	0	0	0	94.93525475	95.03357483	95.12574984	95.21229924	95.29361093	95.36999001	95.44168093	95.5088783	95.5718081	95.63067125	95.68563067	95.73681451	95.7843178	95.82820276	95.86849736	95.90519212	95.93823458	95.96752121	95.99291364	96.01421226	96.03103689	96.04288491	96.04912607	96.04897133	96.04143256	96.02527233	95.99899035	95.9607614	95.90824081	95.83834048	95.74687307	95.6281673	95.48849719	95.33306456	95.13810828	94.89052054	94.57139452	94.15027159	93.57721187	92.76276522	91.52866025	89.44436144	85.31078704	72.83091698	78.4449824	87.30753302	90.7093702	92.49808555	93.59185187	94.32216002	94.83826699	95.21745932	95.38804279	95.7253512	95.89881117	96.06790568	96.19714373	96.29509848	96.36850748	96.4222027	96.45973812	96.48381293	96.49660187	96.49985307	96.49494185	96.48295345	96.4647454	96.4409948	96.41224457	96.37893075	96.34126479	96.29934415	96.25319508	96.20278482	96.14802923	96.08879682	96.02490993	95.95614319	95.88221947	95.80280374	95.71753876	95.62612076	95.52815719	95.42308087	95.31009899	95.18811882	95.05563336	94.91053599	0	0	0	0	0	0	0	0	0	0	0	0	0	0	0	0;
    0	0	0	0	0	0	0	0	0	0	0	0	0	0	0	0	0	0	0	94.9727588	95.07486994	95.16971275	95.2580003	95.34024898	95.41681804	95.48798228	95.55401938	95.61517248	95.67166582	95.72369051	95.77140106	95.81491835	95.85433084	95.88969366	95.9210254	95.94830179	95.97141406	95.98999806	96.00351004	96.01126598	96.01244902	96.00606301	95.99084621	95.96519322	95.92706414	95.87382991	95.80209542	95.70747967	95.58413929	95.42394915	95.2151941	94.94068419	94.57499334	94.07932932	93.48002683	92.62894413	91.34215933	89.1739083	84.87668728	71.92139539	77.84658714	86.94012476	90.4513054	92.3045598	93.44161944	94.19865083	94.80524194	95.24223301	95.56365237	95.80386528	95.98532784	96.12281882	96.22642442	96.30334377	96.35895279	96.39729991	96.42147039	96.43382445	96.43619631	96.43002498	96.41649445	96.39655291	96.37094171	96.34022482	96.30468971	96.26435799	96.21917739	96.16904294	96.11380127	96.05325116	95.98715279	95.91524278	95.83721389	95.75269275	95.6612214	95.56228015	95.45515755	95.33882433	95.21181943	95.07206323	94.91653302	0	0	0	0	0	0	0	0	0	0	0	0	0	0	0	0	0	0	0;
    0	0	0	0	0	0	0	0	0	0	0	0	0	0	0	0	0	0	0	0	0	94.89967847	95.01069778	95.11239453	95.20593511	95.2921491	95.37161922	95.44478389	95.51201006	95.57358523	95.62973738	95.68065165	95.72648321	95.76736691	95.8034139	95.83470162	95.86127158	95.88311058	95.89994734	95.91124559	95.91629727	95.91418912	95.90375505	95.88351358	95.85158576	95.80559161	95.74245993	95.65814642	95.54725145	95.4024387	95.2135151	94.96591712	94.63799166	94.19588153	93.5832965	92.69944725	91.34612096	89.0678572	84.51533276	71.00062319	77.31445609	86.72876714	90.40364233	92.34411255	93.52673145	94.30974645	94.85650189	95.25178313	95.54399028	95.7628655	95.9277899	96.05194173	96.14458171	96.21238744	96.26027404	96.29194914	96.31026896	96.31743311	96.31515106	96.30473972	96.28720586	96.26330527	96.23356425	96.19812591	96.15692114	96.10982729	96.05669017	95.99732808	95.93152012	95.85898944	95.77938047	95.69222285	95.59691854	95.49263946	95.37828116	95.25219496	95.11197699	94.95403519	94.77274949	0	0	0	0	0	0	0	0	0	0	0	0	0	0	0	0	0	0	0	0	0;
    0	0	0	0	0	0	0	0	0	0	0	0	0	0	0	0	0	0	0	0	0	0	0	94.82851518	94.9467397	95.05337946	95.15014127	95.23822406	95.31845293	95.3914419	95.45764431	95.51739292	95.57093086	95.61843864	95.66003272	95.69580417	95.7258107	95.75008653	95.76863742	95.78124632	95.78734244	95.78614034	95.7765919	95.75733695	95.72660729	95.68210663	95.62083687	95.53884312	95.43084033	95.2896943	95.10541311	94.86370085	94.54323513	94.11071773	93.51112037	92.64638936	91.32102515	89.07941602	84.5462282	70.46538904	77.24523472	86.72230163	90.36250494	92.27385594	93.4365152	94.2060115	94.74283853	95.1303728	95.41652273	95.63065139	95.79181616	95.91295807	96.00317325	96.06902388	96.11533772	96.14571774	96.16287318	96.16886003	96.16522347	96.15311891	96.13338191	96.1065208	96.07264227	96.03172079	95.9836848	95.92842439	95.86575047	95.79539211	95.71696277	95.62990661	95.53347181	95.42657721	95.30765972	95.17438354	95.02320786	94.84854291	94.64089571	0	0	0	0	0	0	0	0	0	0	0	0	0	0	0	0	0	0	0	0	0	0	0;
    0	0	0	0	0	0	0	0	0	0	0	0	0	0	0	0	0	0	0	0	0	0	0	0	0	94.76694588	94.88952887	94.99836453	95.09570602	95.18309999	95.2615905	95.3319176	95.39459386	95.44997147	95.4982815	95.53966093	95.57417152	95.60181606	95.62253084	95.63621898	95.6425929	95.64097625	95.63042261	95.60966175	95.57701312	95.5302386	95.46638405	95.38151734	95.27034072	95.12559476	94.93710844	94.69021865	94.36300218	93.9211042	93.30728037	92.41796586	91.04304246	88.67421245	83.75249725	68.59185896	76.17014443	86.18013254	90.01986836	92.00572857	93.20273032	93.99118881	94.53995234	94.93587602	95.22829586	95.44742756	95.61278042	95.7375707	95.8309882	95.89961076	95.94823223	95.9803817	95.99864969	96.0049859	96.00082799	95.9872365	95.96487912	95.9339891	95.89466604	95.84691988	95.7906588	95.72566843	95.65157115	95.56780198	95.47349831	95.36739304	95.247566	95.11106453	94.95325063	94.76645426	94.53668118	0	0	0	0	0	0	0	0	0	0	0	0	0	0	0	0	0	0	0	0	0	0	0	0	0;
    0	0	0	0	0	0	0	0	0	0	0	0	0	0	0	0	0	0	0	0	0	0	0	0	0	0	0	94.71815679	94.8410983	94.94858104	95.04327605	95.1269676	95.20081673	95.26561071	95.32186535	95.36989965	95.40987959	95.44184615	95.4657323	95.48137161	95.48849964	95.48665125	95.47491882	95.4520295	95.41629071	95.36546029	95.29654369	95.20554039	95.08700161	94.93339905	94.73409226	94.47360262	94.12855601	93.66189373	93.01102201	92.06121042	90.57870133	88.01298127	82.71647224	66.46097196	74.95363684	85.41228684	89.48202547	91.59838205	92.8697537	93.70318917	94.28146162	94.69819443	95.00618537	95.2374649	95.41256147	95.54523734	95.64500179	95.71860637	95.77093589	95.80557432	95.82517153	95.83169168	95.82657758	95.81075768	95.78468725	95.74863075	95.70269283	95.64680665	95.58069871	95.50386149	95.41544062	95.31411311	95.19781125	95.06320345	94.90494664	94.71395279	94.47276657	0	0	0	0	0	0	0	0	0	0	0	0	0	0	0	0	0	0	0	0	0	0	0	0	0	0	0;
    0	0	0	0	0	0	0	0	0	0	0	0	0	0	0	0	0	0	0	0	0	0	0	0	0	0	0	0	0	94.68116174	94.79974211	94.90182534	94.99026268	95.06686972	95.13279002	95.18876024	95.23521407	95.27235528	95.30019858	95.31859129	95.32722022	95.32560482	95.31300102	95.28814928	95.24930125	95.19412209	95.11948769	95.02118935	94.89348463	94.72839786	94.51459032	94.23545565	93.86574188	93.36519184	92.66569038	91.64290381	90.0458483	87.28703304	81.6031116	64.18063831	73.6926796	84.59805167	88.89148593	91.13799623	92.49190102	93.38012371	93.99630633	94.44034818	94.76870731	95.015564	95.20276208	95.34486153	95.45189482	95.53095489	95.58715386	95.62422485	95.64491009	95.65121635	95.64448484	95.62549519	95.59473495	95.55243734	95.49856852	95.4328056	95.35444279	95.26225505	95.15424858	95.02716333	94.87558873	94.69019703	94.4528208	0	0	0	0	0	0	0	0	0	0	0	0	0	0	0	0	0	0	0	0	0	0	0	0	0	0	0	0	0;
    0	0	0	0	0	0	0	0	0	0	0	0	0	0	0	0	0	0	0	0	0	0	0	0	0	0	0	0	0	0	94.52069077	94.65116215	94.76053554	94.85307799	94.93144571	94.99727167	95.0515637	95.09488842	95.12748203	95.14931206	95.16010361	95.15934153	95.14624955	95.1196772	95.07784634	95.01831362	94.93778814	94.83181137	94.6942791	94.51667924	94.28686963	93.98701253	93.58992328	93.05223514	92.30067911	91.20199295	89.48807623	86.53157953	80.44915533	61.8246366	72.4324928	83.76938057	88.28427577	90.66058933	92.09803531	93.04321223	93.69975291	94.17329305	94.52374679	94.78744683	94.98760338	95.13966482	95.25425293	95.33885557	95.39884837	95.43813345	95.45954887	95.46505323	95.45588718	95.43285151	95.39636619	95.34647507	95.28278054	95.20434491	95.10949043	94.99541393	94.85731276	94.68678195	94.46776716	94.16236039	0	0	0	0	0	0	0	0	0	0	0	0	0	0	0	0	0	0	0	0	0	0	0	0	0	0	0	0	0	0;
    0	0	0	0	0	0	0	0	0	0	0	0	0	0	0	0	0	0	0	0	0	0	0	0	0	0	0	0	0	0	0	0	94.50438508	94.62044858	94.71610515	94.79499764	94.859287	94.91026727	94.94864531	94.97467908	94.98825364	94.98891147	94.97585051	94.94788076	94.90327324	94.83949595	94.75308227	94.63931141	94.49169049	94.3011422	94.05469946	93.73323703	93.30766913	92.73156863	91.92669998	90.75106182	88.91917019	85.76325581	79.27860546	59.44125217	71.19945031	82.94466451	87.67473846	90.17857387	91.69879138	92.7009958	93.39843101	93.90211149	94.27522452	94.55618946	94.76957449	94.93172798	95.05387512	95.14390962	95.20747467	95.24863707	95.27025767	95.27423319	95.2618083	95.23367636	95.1900025	95.13036874	95.05363912	94.95767458	94.83874645	94.69015864	94.49939521	94.23935627	0	0	0	0	0	0	0	0	0	0	0	0	0	0	0	0	0	0	0	0	0	0	0	0	0	0	0	0	0	0	0	0;
    0	0	0	0	0	0	0	0	0	0	0	0	0	0	0	0	0	0	0	0	0	0	0	0	0	0	0	0	0	0	0	0	0	94.36076575	94.4822049	94.57944864	94.6572182	94.71821411	94.76399226	94.79534581	94.81249329	94.81516895	94.80264896	94.77372479	94.72662226	94.65879036	94.5666011	94.44506897	94.28730702	94.08367071	93.8203365	93.47696784	93.02256738	92.4077784	91.54948251	90.29695374	88.34737004	84.99262007	78.10695184	57.06100682	70.00827782	82.13478103	87.07138317	89.69898563	91.30010647	92.35837811	93.0962449	93.6298908	94.02562333	94.32383874	94.55040688	94.72255099	94.85208767	94.94730583	95.0141008	95.05664231	95.07776432	95.07935642	95.0625396	95.02772371	94.97456429	94.90179573	94.80685525	94.68506121	94.52759778	94.31673761	94.00823092	0	0	0	0	0	0	0	0	0	0	0	0	0	0	0	0	0	0	0	0	0	0	0	0	0	0	0	0	0	0	0	0	0];

    efficiency_map = efficiency_map / 100;
    % 建立插值器（注意维度顺序：行=speed, 列=torque）
    F = griddedInterpolant({speed_rpm, torque_nm}, efficiency_map, ...
                           'linear', 'nearest');  % 插值=linear, 外推=nearest(夹到边界)
    eta = @(spd_rpm, tq_nm) max(0, min(1, F(spd_rpm, tq_nm))); % 顺便夹到[0,1]
    split_grid = 0:0.01:0.99;
    best.split = NaN;
    best.consumption = inf;

    for s = split_grid
        T1_ = s * Torque;
        T2_ = (1-s) * Torque;

        eta1 = eta(spin_1, T1_);
        eta2 = eta(spin_2, T2_);

        P1_loss = pi/30 * T1_ * spin_1 / eta1 * (1 - eta1);
        P2_loss = pi/30 * T2_ * spin_2 / eta2 * (1 - eta2);
        consumption = P1_loss + P2_loss;% the lesser the better

        if consumption < best.consumption
            best.consumption = consumption;
            best.split = s;
        end
    end
    
    split = best.split;
    T1 = best.split * Torque;
    T2 = (1 - best.split) * Torque;
end

== matlab function ModeSwitching/distribute Torque1 ==
  data: Torque input; T1 output; split input; T2 output
function [T1, T2] = fcn(Torque, split)

        T1 = split * Torque;
        T2 = (1 - split) * Torque;
    end

== matlab function ModeSwitching/Based on economic execution/MATLAB Function ==
  data: T1_dis input; y1 output; y2 output; T2_dis input; eta1 input; eta2 input; eta3 input; moto_spin_1 input; moto_spin_2 input
function [y1, y2] = fcn(T1_dis, T2_dis, eta1, eta2, eta3, moto_spin_1, moto_spin_2)

T_total = T1_dis + T2_dis;
P1_loss = T1_dis * moto_spin_1 / eta1 * (1 - eta1);
P2_loss = T2_dis * moto_spin_2 / eta2 * (1 - eta2);
P_loss = T_total * (moto_spin_1 + moto_spin_2) /2 / eta3 * (1 - eta3);
if P1_loss+P2_loss < P_loss
    y1 = T1_dis;
    y2 = T2_dis;
else
    y1 = 0;
    y2 = T_total;
end

== matlab function ModeSwitching/Based on economic execution/MATLAB Function1 ==
  data: u1 input; y output; u2 input
function y = fcn(u1, u2)

y = (u1+u2)/2;
